simulink model "Senorless"  (R2023a)
settings: Solver=FixedStepDiscrete  StartTime=0.0  StopTime=5  FixedStep=1/FOC_FRQ  RelTol=1e-3
values from neighbouring files (symbols this model uses):
  ADC_REF = 3.6    [Senorless.sldd]
  ADC_SAMPLE_MAX = 32767.0    [Senorless.sldd]
  AMP_GAIN = 16.0    [Senorless.sldd]
  CURR_INPUT = 3276.0    [Senorless.sldd]
  CURR_KI = 380.0    [Senorless.sldd]
  CURR_KP = 0.04    [Senorless.sldd]
  CURR_LIMIT = 0.95    [Senorless.sldd]
  CURR_OVER = 6.0    [Senorless.sldd]
  CURR_POINT_GAIN = 7.0    [Senorless.sldd]
  CURR_STEP = 32760.0    [Senorless.sldd]
  CURR_UNDER = 0.03    [Senorless.sldd]
  CURR_WIDTH = 6552.0    [Senorless.sldd]
  FOC_FRQ = 25000.0    [Senorless.sldd]
  GAMMA = 32767.0    [Senorless.sldd]
  IMAX = 10.0    [Senorless.sldd]
  LPF_FRQ = 2000.0    [Senorless.sldd]
  MOTOR_DAMPER = 2.06E-7    [Senorless.sldd]
  MOTOR_FLUX = 0.00212352    [Senorless.sldd]
  MOTOR_INERTIA = 4.0E-7    [Senorless.sldd]
  MOTOR_LS = 0.000536    [Senorless.sldd]
  MOTOR_PN = 7.0    [Senorless.sldd]
  MOTOR_RS = 4.0    [Senorless.sldd]
  OPEN_IQ = 0.28    [Senorless.sldd]
  OPEN_IQ_MIN = 0.05    [Senorless.sldd]
  OPEN_IQ_SLOW = 0.1    [Senorless.sldd]
  OPEN_SPD = 1000.0    [Senorless.sldd]
  OPEN_SPD_SLOW = 180.0    [Senorless.sldd]
  OPEN_TIME = 0.5    [Senorless.sldd]
  OPEN_TIME_NFO = 0.5    [Senorless.sldd]
  PLL_LIMIT = 0.9    [Senorless.sldd]
  PLL_WIDTH = 800.0    [Senorless.sldd]
  PWM_FRQ = 96000000.0    [Senorless.sldd]
  RS_HUNT = 0.02    [Senorless.sldd]
  SMOK_FRQ = 600.0    [Senorless.sldd]
  SPD_LIMIT = 0.9    [Senorless.sldd]
  SPD_LPF_LEVEL = 0.0    [Senorless.sldd]
  SPD_MAX = 12000.0    [Senorless.sldd]
  SPD_MIN = 4000.0    [Senorless.sldd]
  SPD_REDUCE = 380.0    [Senorless.sldd]
  SPD_STEP = 6.0    [Senorless.sldd]
  SPD_WIDTH = 20.0    [Senorless.sldd]
  THETA_ERR_LIMIT = 8192.0    [Senorless.sldd]
  TS_POINT_GAIN = 10.0    [Senorless.sldd]
  UDC = 48.0    [Senorless.sldd]
  UDC_GAIN = 21.0    [Senorless.sldd]
  UDC_POINT_GAIN = 10.0    [Senorless.sldd]
undefined symbols (not defined in the file or in its folder): curr_q_ki, curr_q_kp, DiscIntNeverNeededParam, magnitude, PLL_LPF_LEVEL, Udc
libraries: simulink x20, slpidlib x5, mcbcontrolslib x2, mcbplantlib x1, autolibpmsmexterior x1, spspowerguiLib x1
(part 4 of 8)

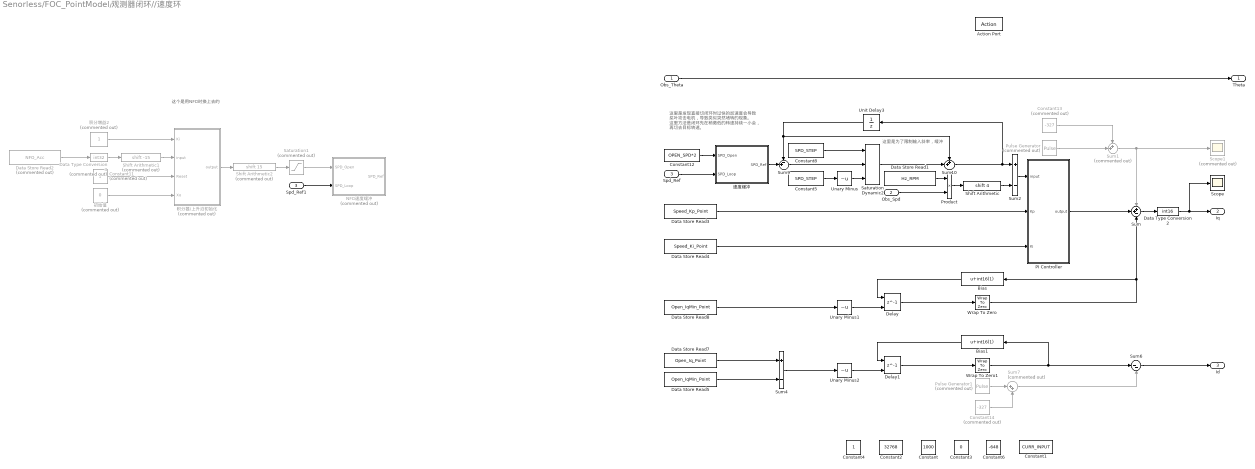
== system Senorless/FOC_PointModel/观测器闭环//速度环 ==
  note: 这个是用NFO时换上去的
  note: 这里是发现直接切闭环时过快的加速度会导致
      | 桨叶攻击电机，导致类似突然堵转的现象。
      | 这里方法是闭环先在稍微低的转速持续一小会，
      | 再切去目标转速。
  note: 这里是为了限制输入斜率，缓冲
  Obs_Theta : Inport
  Obs_Spd : Inport  Port=2
  Spd_Ref : Inport  Port=3
  Action Port : ActionPort  InitializeStates=reset  ActionPortLabel=case [ 4 ]:
  Bias : Bias  Bias=int16(1)  SaturateOnIntegerOverflow=off
  Bias1 : Bias  Bias=int16(1)  SaturateOnIntegerOverflow=off
  Constant : Constant  Value=1000  OutDataTypeStr=int16
  Constant1 : Constant  Value=CURR_INPUT  OutDataTypeStr=int16
  Constant11 : Constant  Commented=on  OutDataTypeStr=uint8
  Constant12 : Constant  Value=OPEN_SPD*2  OutDataTypeStr=int32
  Constant13 : Constant  Commented=on  Value=-327  OutDataTypeStr=int32
  Constant14 : Constant  Commented=on  Value=-327  OutDataTypeStr=int16
  Constant2 : Constant  Value=32768  OutDataTypeStr=int16
  Constant3 : Constant  Value=0  OutDataTypeStr=int16
  Constant4 : Constant  OutDataTypeStr=int16
  Constant5 : Constant  Value=SPD_STEP  OutDataTypeStr=int32
  Constant6 : Constant  Value=-648  OutDataTypeStr=int16
  Constant8 : Constant  Value=SPD_STEP  OutDataTypeStr=int32
  Data Store Read1 : DataStoreRead  DataStoreName=Hz_RPM  IndexOptions=Index vector (dialog)  Indices=1  OutputSizes=1
  Data Store Read2 : DataStoreRead  Commented=on  DataStoreName=NFO_Acc  IndexOptions=Index vector (dialog)  Indices=1  OutputSizes=1
  Data Store Read3 : DataStoreRead  DataStoreName=Speed_Kp_Point  IndexOptions=Index vector (dialog)  Indices=1  OutputSizes=1
  Data Store Read4 : DataStoreRead  DataStoreName=Speed_Ki_Point  IndexOptions=Index vector (dialog)  Indices=1  OutputSizes=1
  Data Store Read5 : DataStoreRead  DataStoreName=Open_IqMin_Point  IndexOptions=Index vector (dialog)  Indices=1  OutputSizes=1
  Data Store Read7 : DataStoreRead  DataStoreName=Open_Iq_Point  IndexOptions=Index vector (dialog)  Indices=1  OutputSizes=1
  Data Store Read8 : DataStoreRead  DataStoreName=Open_IqMin_Point  IndexOptions=Index vector (dialog)  Indices=1  OutputSizes=1
  Data Type Conversion2 : DataTypeConversion  OutDataTypeStr=int16  SaturateOnIntegerOverflow=off
  Data Type Conversion3 : DataTypeConversion  Commented=on  OutDataTypeStr=int32  SaturateOnIntegerOverflow=off
  Delay : Delay  DelayLength=1  InitialConditionSource=Input port
      settings: InputPortMap=u0,p4
  Delay1 : Delay  DelayLength=1  InitialConditionSource=Input port
      settings: InputPortMap=u0,p4
  NFO速度缓冲 : Stateflow chart  Commented=on  TreatAsAtomicUnit=on
  PI Controller : Subsystem
      settings: MinAlgLoopOccurrences=on
  Product : Product  OutDataTypeStr=int32  RndMeth=Zero
  Pulse Generator : DiscretePulseGenerator  Commented=on  Amplitude=int32(654)  Period=1000  PulseWidth=500  SampleTime=-1
  Pulse Generator1 : DiscretePulseGenerator  Commented=on  Amplitude=int16(327*2)  Period=500  PulseWidth=250  SampleTime=-1
  Saturation Dynamic2 : simulink/Discontinuities/Saturation Dynamic  OutMin=[]  OutMax=[]  OutDataTypeStr=Inherit: Same as second input  OutDataType=fixdt(1, 16)  OutScaling=2^-10  RndMeth=Zero  DoSatur=off
  Saturation1 : Saturate  Commented=on  UpperLimit=SPD_MIN  LowerLimit=0
  Scope : Scope
  Scope1 : Scope  Commented=on
  Shift Arithmetic : ArithShift  BitShiftNumber=4
  Shift Arithmetic1 : ArithShift  Commented=on  BitShiftNumber=-15
  Shift Arithmetic2 : ArithShift  Commented=on  BitShiftNumber=15
  Spd_Ref1 : InportShadow  Port=3
  Sum : Sum  Inputs=++-  RndMeth=Zero
  Sum1 : Sum  Commented=on  Inputs=++|  RndMeth=Zero
  Sum10 : Sum  Inputs=++|  OutDataTypeStr=int32  RndMeth=Zero
  Sum2 : Sum  Inputs=+-  AccumDataTypeStr=int32  OutDataTypeStr=int16  RndMeth=Zero  SaturateOnIntegerOverflow=on
  Sum4 : Sum  Inputs=+-
  Sum6 : Sum  Inputs=|--  OutDataTypeStr=int16  RndMeth=Zero
  Sum7 : Sum  Commented=on  Inputs=|++  RndMeth=Zero
  Sum9 : Sum  Inputs=-+|  AccumDataTypeStr=int16  OutDataTypeStr=int32  RndMeth=Zero
  Unary Minus : UnaryMinus
  Unary Minus1 : UnaryMinus
  Unary Minus2 : UnaryMinus
  Unit Delay3 : UnitDelay  InitialCondition=OPEN_SPD  SampleTime=-1  HasFrameUpgradeWarning=on
  Wrap To Zero : simulink/Discontinuities/Wrap To Zero  Threshold=int16(0)
  Wrap To Zero1 : simulink/Discontinuities/Wrap To Zero  Threshold=int16(0)
  初始值 : Constant  Commented=on  Value=0  OutDataTypeStr=int32
  积分器/上升沿初始化 : Subsystem  Commented=on  TreatAsAtomicUnit=on
      settings: MinAlgLoopOccurrences=on
  积分增益2 : Constant  Commented=on  OutDataTypeStr=int16
  速度缓冲 : Stateflow chart  TreatAsAtomicUnit=on
  Theta : Outport
  Iq : Outport  Port=2
  Id : Outport  Port=3
  wires:
  Obs_Theta/1 -> Theta/1
  Data Store Read4/1 -> PI Controller/3(Ki)
  Data Store Read3/1 -> PI Controller/2(Kp)
  Sum10/1 -> Unit Delay3/1, Sum2/1
  Sum2/1 -> PI Controller/1(input)
  Shift Arithmetic/1 -> Sum2/2
  Data Store Read1/1 -> Product/1
  Obs_Spd/1 -> Product/2
  Saturation Dynamic2/1 -> Sum10/2
  Unit Delay3/1 -> Sum10/1, Sum9/1
  Data Store Read7/1 -> Sum4/1
  Spd_Ref/1 -> 速度缓冲/2(SPD_Loop)
  Product/1 -> Shift Arithmetic/1
  PI Controller/1(output) -> Sum/2
  Sum/1 -> Data Type Conversion2/1
  Constant5/1 -> Unary Minus/1
  积分器/上升沿初始化/1(output) -> Shift Arithmetic2/1
  Data Store Read2/1 -> Data Type Conversion3/1
  积分增益2/1 -> 积分器/上升沿初始化/1(Ki)
  Data Type Conversion3/1 -> Shift Arithmetic1/1
  Shift Arithmetic1/1 -> 积分器/上升沿初始化/2(input)
  Constant12/1 -> 速度缓冲/1(SPD_Open)
  Spd_Ref1/1 -> NFO速度缓冲/2(SPD_Loop)
  Shift Arithmetic2/1 -> Saturation1/1
  Constant11/1 -> 积分器/上升沿初始化/3(Reset)
  初始值/1 -> 积分器/上升沿初始化/4(Xo)
  Saturation1/1 -> NFO速度缓冲/1(SPD_Open)
  速度缓冲/1(SPD_Ref) -> Sum9/2
  Data Store Read5/1 -> Sum4/2
  Data Type Conversion2/1 -> Iq/1, Scope/1
  Sum1/1 -> Sum/1, Scope1/1
  Sum6/1 -> Id/1
  Pulse Generator1/1 -> Sum7/1
  Constant14/1 -> Sum7/2
  Sum7/1 -> Sum6/2
  Sum9/1 -> Saturation Dynamic2/2
  Constant8/1 -> Saturation Dynamic2/1
  Unary Minus/1 -> Saturation Dynamic2/3
  Pulse Generator/1 -> Sum1/2
  Constant13/1 -> Sum1/1
  Sum4/1 -> Unary Minus2/1
  Delay/1 -> Wrap To Zero/1
  Data Store Read8/1 -> Unary Minus1/1
  Unary Minus1/1 -> Delay/2
  Wrap To Zero/1 -> Bias/1, Sum/3
  Unary Minus2/1 -> Delay1/2
  Delay1/1 -> Wrap To Zero1/1
  Wrap To Zero1/1 -> Sum6/1, Bias1/1
  Bias1/1 -> Delay1/1
  Bias/1 -> Delay/1

== system Senorless/FOC_PointModel/预定位 ==
  Action Port : ActionPort  InitializeStates=reset  ActionPortLabel=case [ 1 ]:
  Bias : Bias  Bias=int16(5)  SaturateOnIntegerOverflow=off
  Constant1 : Constant  Value=0  OutDataTypeStr=int16
  Constant2 : Constant  OutDataTypeStr=int16
  Constant3 : Constant  Value=0  OutDataTypeStr=uint16
  Data Store Read3 : DataStoreRead  DataStoreName=Open_Iq_Point  IndexOptions=Index vector (dialog)  Indices=1  OutputSizes=1
  Saturation Dynamic2 : simulink/Discontinuities/Saturation Dynamic  OutMin=[]  OutMax=[]  OutDataTypeStr=Inherit: Same as second input  OutDataType=fixdt(1, 16)  OutScaling=2^-10  RndMeth=Zero  DoSatur=off
  Unit Delay4 : UnitDelay  SampleTime=-1  HasFrameUpgradeWarning=on
  Theta : Outport
  Iq : Outport  Port=2
  Id : Outport  Port=3
  wires:
  Constant3/1 -> Theta/1
  Constant1/1 -> Iq/1
  Saturation Dynamic2/1 -> Unit Delay4/1, Id/1
  Constant2/1 -> Saturation Dynamic2/3
  Bias/1 -> Saturation Dynamic2/2
  Data Store Read3/1 -> Saturation Dynamic2/1
  Unit Delay4/1 -> Bias/1

== system Senorless/FOC_PointModel/Err/PLL_LPF1 ==
  note: y(n)=ax(n)+(1−a)y(n−1)
  note: a =(ω c​ T s​ )/(1+ω c​ T s​ )
  input : Inport
  Constant1 : Constant  Value=15  OutDataTypeStr=int16
  Constant5 : Constant  OutDataTypeStr=int16
  Product10 : Product  OutDataTypeStr=int32
  Product11 : Product  OutDataTypeStr=int32  RndMeth=Zero
  Shift Arithmetic1 : ArithShift  BitShiftNumber=-4
  Shift Arithmetic9 : ArithShift  BitShiftNumber=4
  Sum10 : Sum  Inputs=-+
  Sum11 : Sum  OutDataTypeStr=int32  RndMeth=Zero
  Unit Delay9 : UnitDelay  SampleTime=-1  HasFrameUpgradeWarning=on
  output : Outport
  wires:
  input/1 -> Product10/2
  Unit Delay9/1 -> Product11/1
  Product10/1 -> Sum11/2
  Product11/1 -> Sum11/1
  Sum10/1 -> Product10/1
  Shift Arithmetic1/1 -> Sum10/2
  Shift Arithmetic9/1 -> Unit Delay9/1, output/1
  Sum11/1 -> Shift Arithmetic9/1
  Constant5/1 -> Shift Arithmetic1/1
  Constant1/1 -> Product11/2, Sum10/1

== system Senorless/FOC_PointModel/Err/闭环错误判断 ==
  Curr_Err : Inport
  Curr_Max : Inport  Port=2
  Obs_SPD : Inport  Port=3
  Udc_Ref : Inport  Port=4
  Enable : EnablePort  StatesWhenEnabling=reset
  Constant : Constant  Value=16384  OutDataTypeStr=int32
  Data Store Read : DataStoreRead  DataStoreName=FOC_FRQ_Point  IndexOptions=Index vector (dialog)  Indices=1  OutputSizes=1
  Data Store Read4 : DataStoreRead  DataStoreName=Open_Hz  IndexOptions=Index vector (dialog)  Indices=1  OutputSizes=1
  Data Store Read7 : DataStoreRead  DataStoreName=Curr_Under  IndexOptions=Index vector (dialog)  Indices=1  OutputSizes=1
  Data Type Conversion12 : DataTypeConversion  OutDataTypeStr=int32  SaturateOnIntegerOverflow=off
  Data Type Conversion13 : DataTypeConversion  OutDataTypeStr=uint8  SaturateOnIntegerOverflow=off
  If1 : If
  Logical Operator : Logic  Operator=OR  Inputs=3  AllPortsSameDT=off  OutDataTypeStr=boolean
  Merge3 : Merge
  OR1 : Logic  Operator=OR  AllPortsSameDT=off  OutDataTypeStr=boolean
  Relational Operator1 : RelationalOperator  Operator=<  OutDataTypeStr=boolean  RndMeth=Zero  InputSameDT=off
  Relational Operator2 : RelationalOperator  Operator=<  OutDataTypeStr=boolean  RndMeth=Zero  InputSameDT=off
  Relational Operator3 : RelationalOperator  OutDataTypeStr=boolean  RndMeth=Zero  InputSameDT=off
  Relational Operator4 : RelationalOperator  Operator=<  OutDataTypeStr=boolean  RndMeth=Zero  InputSameDT=off
  SUM : Subsystem
  Scope : Scope
  Scope1 : Scope
  Scope2 : Scope
  Shift Arithmetic1 : ArithShift  BitShiftNumber=1
  Shift Arithmetic3 : ArithShift  BitShiftNumber=1
  Unit Delay : UnitDelay  SampleTime=-1  HasFrameUpgradeWarning=on
  ZERO : Subsystem
  Run_Err : Outport
  wires:
  If1/2 -> ZERO/Action
  Data Store Read/1 -> Shift Arithmetic1/1
  Data Store Read7/1 -> Relational Operator1/2
  Data Type Conversion12/1 -> SUM/1(in)
  Data Store Read4/1 -> Shift Arithmetic3/1
  Logical Operator/1 -> Data Type Conversion12/1, Data Type Conversion13/1
  ZERO/1(out) -> Merge3/2
  Relational Operator3/1 -> Scope2/1, OR1/2
  Curr_Max/1 -> Relational Operator1/1
  Curr_Err/1 -> OR1/1
  If1/1 -> SUM/Action
  Shift Arithmetic3/1 -> Relational Operator2/2
  Merge3/1 -> Scope1/1, Relational Operator3/1
  OR1/1 -> Scope/1, Run_Err/1
  Data Type Conversion13/1 -> If1/1
  SUM/1(out) -> Merge3/1
  Shift Arithmetic1/1 -> Relational Operator3/2
  Relational Operator2/1 -> Logical Operator/3
  Relational Operator1/1 -> Logical Operator/2
  Relational Operator4/1 -> Logical Operator/1
  Constant/1 -> Relational Operator4/2
  Udc_Ref/1 -> Relational Operator4/1
  Obs_SPD/1 -> Unit Delay/1
  Unit Delay/1 -> Relational Operator2/1

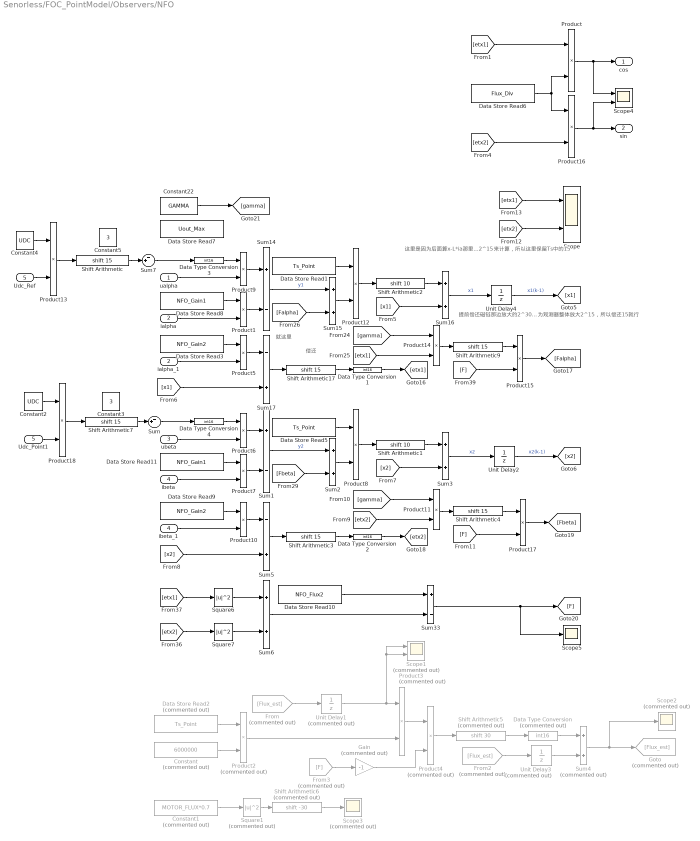
== system Senorless/FOC_PointModel/Observers/NFO ==
  note: 提前偿还磁链那边放大的2^30，因为观测器整体放大2^15，所以偿还15就行
  note: 偿还
  note: 就这里
  note: 这里是因为后面算x-L*ia那里需要再放大2^15来计算，所以这里保留Ts中的15
  ualpha : Inport
  ialpha : Inport  Port=2
  ubeta : Inport  Port=3
  ibeta : Inport  Port=4
  Udc_Ref : Inport  Port=5
  Constant : Constant  Commented=on  Value=6000000  OutDataTypeStr=int32
  Constant1 : Constant  Commented=on  Value=MOTOR_FLUX*0.7  OutDataTypeStr=single
  Constant2 : Constant  Value=UDC  OutDataTypeStr=int16
  Constant22 : Constant  Value=GAMMA  OutDataTypeStr=uint32
  Constant3 : Constant  Value=3  OutDataTypeStr=int16
  Constant4 : Constant  Value=UDC  OutDataTypeStr=int16
  Constant5 : Constant  Value=3  OutDataTypeStr=int16
  Data Store Read1 : DataStoreRead  DataStoreName=Ts_Point  IndexOptions=Index vector (dialog)  Indices=1  OutputSizes=1
  Data Store Read10 : DataStoreRead  DataStoreName=NFO_Flux2  IndexOptions=Index vector (dialog)  Indices=1  OutputSizes=1
  Data Store Read11 : DataStoreRead  DataStoreName=NFO_Gain1  IndexOptions=Index vector (dialog)  Indices=1  OutputSizes=1
  Data Store Read2 : DataStoreRead  Commented=on  DataStoreName=Ts_Point  IndexOptions=Index vector (dialog)  Indices=1  OutputSizes=1
  Data Store Read3 : DataStoreRead  DataStoreName=NFO_Gain2  IndexOptions=Index vector (dialog)  Indices=1  OutputSizes=1
  Data Store Read5 : DataStoreRead  DataStoreName=Ts_Point  IndexOptions=Index vector (dialog)  Indices=1  OutputSizes=1
  Data Store Read6 : DataStoreRead  DataStoreName=Flux_Div  IndexOptions=Index vector (dialog)  Indices=1  OutputSizes=1
  Data Store Read7 : DataStoreRead  DataStoreName=Uout_Max  IndexOptions=Index vector (dialog)  Indices=1  OutputSizes=1
  Data Store Read8 : DataStoreRead  DataStoreName=NFO_Gain1  IndexOptions=Index vector (dialog)  Indices=1  OutputSizes=1
  Data Store Read9 : DataStoreRead  DataStoreName=NFO_Gain2  IndexOptions=Index vector (dialog)  Indices=1  OutputSizes=1
  Data Type Conversion : DataTypeConversion  Commented=on  OutDataTypeStr=int16  SaturateOnIntegerOverflow=off
  Data Type Conversion{1..4} (4 alike) : DataTypeConversion  OutDataTypeStr=int16  SaturateOnIntegerOverflow=off
  From : From  Commented=on  GotoTag=Flux_est
  From2 : From  Commented=on  GotoTag=Flux_est
  From3 : From  Commented=on  GotoTag=F
  Gain : Gain  Commented=on  Gain=-1  OutDataTypeStr=int16  RndMeth=Zero
  Goto : Goto  Commented=on  GotoTag=Flux_est
  Product : Product
  Product{1,5..12,14..15,17} (12 alike) : Product  OutDataTypeStr=int32  RndMeth=Zero
  Product13 : Product  OutDataTypeStr=int32
  Product16 : Product
  Product18 : Product  OutDataTypeStr=int32
  Product2 : Product  Commented=on  OutDataTypeStr=int32  RndMeth=Zero
  Product3 : Product  Commented=on  OutDataTypeStr=int32  RndMeth=Zero
  Product4 : Product  Commented=on  OutDataTypeStr=int32  RndMeth=Zero
  Scope : Scope  NumInputPorts=2
  Scope1 : Scope  Commented=on  NumInputPorts=2
  Scope2 : Scope  Commented=on
  Scope3 : Scope  Commented=on
  Scope4 : Scope  NumInputPorts=2
  Scope5 : Scope
  Shift Arithmetic{,3..4,7,9,17} (6 alike) : ArithShift  BitShiftNumber=15
  Shift Arithmetic1 : ArithShift  BitShiftNumber=10
  Shift Arithmetic2 : ArithShift  BitShiftNumber=10
  Shift Arithmetic5 : ArithShift  Commented=on  BitShiftNumber=30
  Shift Arithmetic6 : ArithShift  Commented=on  BitShiftNumber=-30
  Square1 : Math  Commented=on  Operator=magnitude^2
  Square6 : Math  Operator=magnitude^2
  Square7 : Math  Operator=magnitude^2
  Sum : Sum  Inputs=-+|
  Sum1 : Sum  Inputs=+-  OutDataTypeStr=int32  RndMeth=Zero
  Sum14 : Sum  Inputs=+-  OutDataTypeStr=int32  RndMeth=Zero
  Sum{2..3,6,15..16} (5 alike) : Sum  OutDataTypeStr=int32  RndMeth=Zero
  Sum17 : Sum  Inputs=-+  OutDataTypeStr=int32  RndMeth=Zero
  Sum33 : Sum  Inputs=+-  OutDataTypeStr=int16  RndMeth=Zero
  Sum4 : Sum  Commented=on  OutDataTypeStr=int16  RndMeth=Zero
  Sum5 : Sum  Inputs=-+  OutDataTypeStr=int32  RndMeth=Zero
  Sum7 : Sum  Inputs=-+|
  Udc_Point1 : InportShadow  Port=5
  Unit Delay1 : UnitDelay  Commented=on  SampleTime=-1  HasFrameUpgradeWarning=on
  Unit Delay2 : UnitDelay  SampleTime=-1  HasFrameUpgradeWarning=on
  Unit Delay3 : UnitDelay  Commented=on  InitialCondition=4842  SampleTime=-1  HasFrameUpgradeWarning=on
  Unit Delay4 : UnitDelay  SampleTime=-1  HasFrameUpgradeWarning=on
  ialpha_1 : InportShadow  Port=2
  ibeta_1 : InportShadow  Port=4
  cos : Outport
  sin : Outport  Port=2
  wires:
  Sum3/1 -> Unit Delay2/1  "x2"
  [gamma] -> Product14/1
  Product17/1 -> [Fbeta]
  Unit Delay2/1 -> [x2]  "x2(k-1)"
  Data Store Read1/1 -> Product12/1
  [etx1] -> Scope/1
  [x1] -> Sum16/2
  Data Store Read9/1 -> Product10/1
  ialpha_1/1 -> Product5/2
  Product1/1 -> Sum14/2
  [x2] -> Sum5/2
  Constant22/1 -> [gamma]
  Shift Arithmetic4/1 -> Product17/1
  ubeta/1 -> Product6/2
  Sum6/1 -> Sum33/2
  Sum15/1 -> Product12/2
  Product12/1 -> Shift Arithmetic2/1
  Sum2/1 -> Product8/2
  Product8/1 -> Shift Arithmetic1/1
  [gamma] -> Product11/1
  [x2] -> Sum3/2
  ibeta/1 -> Product7/2
  Square6/1 -> Sum6/1
  Product7/1 -> Sum1/2
  Sum17/1 -> Shift Arithmetic17/1
  Data Store Read5/1 -> Product8/1
  ialpha/1 -> Product1/2
  [etx2] -> Scope/2
  Sum5/1 -> Shift Arithmetic3/1
  ualpha/1 -> Product9/2
  [F] -> Product17/2
  [Falpha] -> Sum15/2
  Product10/1 -> Sum5/1
  Product11/1 -> Shift Arithmetic4/1
  Sum16/1 -> Unit Delay4/1  "x1"
  Product5/1 -> Sum17/1
  Data Store Read8/1 -> Product1/1
  [etx2] -> Square7/1
  [etx2] -> Product11/2
  [Fbeta] -> Sum2/2
  Shift Arithmetic2/1 -> Sum16/1
  Unit Delay4/1 -> [x1]  "x1(k-1)"
  Product15/1 -> [Falpha]
  [etx1] -> Product14/2
  [etx1] -> Square6/1
  Shift Arithmetic3/1 -> Data Type Conversion2/1
  Shift Arithmetic1/1 -> Sum3/1
  [x1] -> Sum17/2
  ibeta_1/1 -> Product10/2
  Data Store Read11/1 -> Product7/1
  Sum14/1 -> Sum15/1  "y1"
  Shift Arithmetic17/1 -> Data Type Conversion1/1
  Sum1/1 -> Sum2/1  "y2"
  Data Store Read3/1 -> Product5/1
  Square7/1 -> Sum6/2
  Constant/1 -> Product2/2
  Data Store Read2/1 -> Product2/1
  Sum33/1 -> Scope5/1, [F]
  From3/1 -> Gain/1
  Product4/1 -> Shift Arithmetic5/1
  Unit Delay1/1 -> Scope1/2, Scope1/1, Product3/1
  From/1 -> Unit Delay1/1
  Product3/1 -> Product4/1
  Shift Arithmetic5/1 -> Data Type Conversion/1
  Gain/1 -> Product4/2
  Data Type Conversion/1 -> Sum4/1
  Unit Delay3/1 -> Sum4/2
  Sum4/1 -> Goto/1, Scope2/1
  From2/1 -> Unit Delay3/1
  Product2/1 -> Product3/2
  Constant1/1 -> Square1/1
  Square1/1 -> Shift Arithmetic6/1
  Shift Arithmetic6/1 -> Scope3/1
  Data Store Read10/1 -> Sum33/1
  Data Store Read6/1 -> Product16/1, Product/2
  Product/1 -> cos/1, Scope4/1
  Product16/1 -> sin/1, Scope4/2
  Product14/1 -> Shift Arithmetic9/1
  Data Type Conversion1/1 -> [etx1]
  Shift Arithmetic9/1 -> Product15/1
  [F] -> Product15/2
  Data Type Conversion2/1 -> [etx2]
  [etx1] -> Product/1
  [etx2] -> Product16/2
  Product13/1 -> Shift Arithmetic/1
  Constant4/1 -> Product13/1
  Udc_Ref/1 -> Product13/2
  Constant2/1 -> Product18/1
  Product18/1 -> Shift Arithmetic7/1
  Udc_Point1/1 -> Product18/2
  Product9/1 -> Sum14/1
  Product6/1 -> Sum1/1
  Data Type Conversion3/1 -> Product9/1
  Shift Arithmetic7/1 -> Sum/2
  Data Type Conversion4/1 -> Product6/1
  Sum/1 -> Data Type Conversion4/1
  Shift Arithmetic/1 -> Sum7/2
  Sum7/1 -> Data Type Conversion3/1

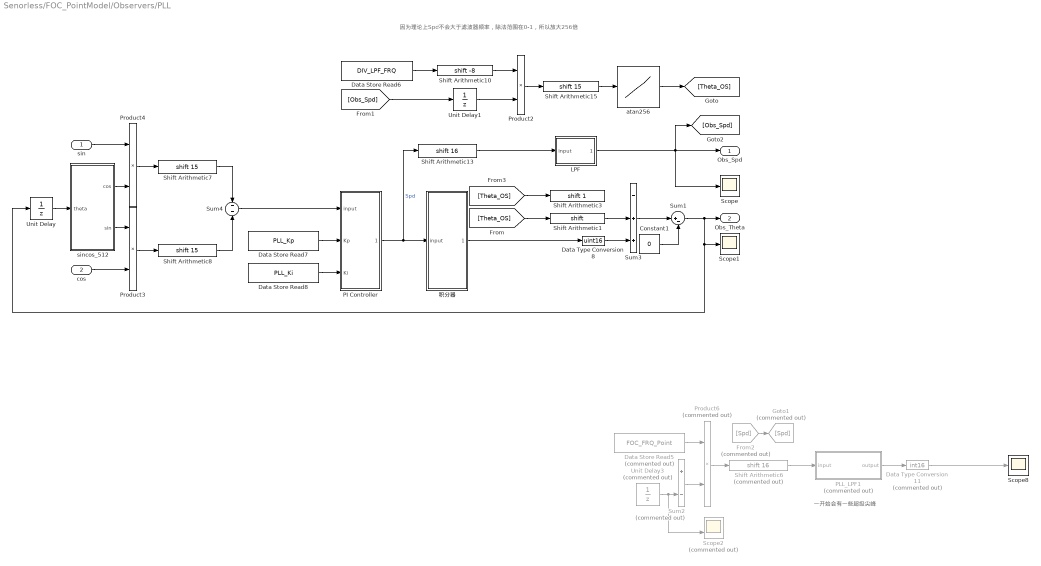
== system Senorless/FOC_PointModel/Observers/PLL ==
  note: 一开始会有一些超级尖峰
  note: 因为理论上Spd不会大于滤波器频率，除法范围在0-1，所以放大256倍
  sin : Inport
  cos : Inport  Port=2
  Constant1 : Constant  Value=0  OutDataTypeStr=uint16
  Data Store Read5 : DataStoreRead  Commented=on  DataStoreName=FOC_FRQ_Point  IndexOptions=Index vector (dialog)  Indices=1  OutputSizes=1
  Data Store Read6 : DataStoreRead  DataStoreName=DIV_LPF_FRQ  IndexOptions=Index vector (dialog)  Indices=1  OutputSizes=1
  Data Store Read7 : DataStoreRead  DataStoreName=PLL_Kp  IndexOptions=Index vector (dialog)  Indices=1  OutputSizes=1
  Data Store Read8 : DataStoreRead  DataStoreName=PLL_Ki  IndexOptions=Index vector (dialog)  Indices=1  OutputSizes=1
  Data Type Conversion11 : DataTypeConversion  Commented=on  OutDataTypeStr=int16  SaturateOnIntegerOverflow=off
  Data Type Conversion8 : DataTypeConversion  OutDataTypeStr=uint16  SaturateOnIntegerOverflow=off
  From2 : From  Commented=on  GotoTag=Spd
  Goto1 : Goto  Commented=on  GotoTag=Spd
  LPF : Subsystem  TreatAsAtomicUnit=on
  PI Controller : Subsystem
      settings: MinAlgLoopOccurrences=on
  PLL_LPF1 : Subsystem  Commented=on  TreatAsAtomicUnit=on
  Product2 : Product  OutDataTypeStr=int32  RndMeth=Zero
  Product3 : Product  OutDataTypeStr=int32  RndMeth=Zero
  Product4 : Product  OutDataTypeStr=int32  RndMeth=Zero
  Product6 : Product  Commented=on  OutDataTypeStr=int32  RndMeth=Zero
  Scope : Scope
  Scope1 : Scope
  Scope2 : Scope  Commented=on  NumInputPorts=2
  Scope8 : Scope
  Shift Arithmetic1 : ArithShift
  Shift Arithmetic10 : ArithShift  BitShiftNumber=-8
  Shift Arithmetic13 : ArithShift  BitShiftNumber=16
  Shift Arithmetic15 : ArithShift  BitShiftNumber=15
  Shift Arithmetic3 : ArithShift  BitShiftNumber=1
  Shift Arithmetic6 : ArithShift  Commented=on  BitShiftNumber=16
  Shift Arithmetic7 : ArithShift  BitShiftNumber=15
  Shift Arithmetic8 : ArithShift  BitShiftNumber=15
  Sum1 : Sum  Inputs=|+-  AccumDataTypeStr=uint16  OutDataTypeStr=uint16  RndMeth=Zero
  Sum2 : Sum  Commented=on  Inputs=+-  OutDataTypeStr=int16  RndMeth=Zero
  Sum3 : Sum  Inputs=-++  AccumDataTypeStr=uint16  OutDataTypeStr=uint16  RndMeth=Zero
  Sum4 : Sum  Inputs=--
  Unit Delay : UnitDelay  SampleTime=-1  HasFrameUpgradeWarning=on
  Unit Delay1 : UnitDelay  SampleTime=-1  HasFrameUpgradeWarning=on
  Unit Delay3 : UnitDelay  Commented=on  SampleTime=-1  HasFrameUpgradeWarning=on
  atan256 : Lookup_n-D  NumberOfTableDimensions=1  BreakpointsSpecification=Even spacing  BreakpointsForDimension1=[-5:5]  UseOneInputPortForAllInputData=on  Table=uint16(16384*atan(linspace(0,1,256)))  TableDataTypeStr=uint16  InterpMethod=Flat  RemoveProtectionInput=on  InternalRulePriority=Speed  OutDataTypeStr=uint16  RndMeth=Zero
  sincos_512 : Subsystem
  积分器 : Subsystem
      settings: MinAlgLoopOccurrences=on
  Obs_Spd : Outport
  Obs_Theta : Outport  Port=2
  wires:
  Data Store Read8/1 -> PI Controller/3(Ki)
  From2/1 -> Goto1/1
  Sum2/1 -> Product6/2
  Unit Delay3/1 -> Scope2/2, Sum2/2
  Product6/1 -> Shift Arithmetic6/1
  Data Store Read5/1 -> Product6/1
  Data Store Read7/1 -> PI Controller/2(Kp)
  积分器/1(output) -> Data Type Conversion8/1
  Shift Arithmetic6/1 -> PLL_LPF1/1(input)
  Sum3/1 -> Sum1/1
  Data Type Conversion8/1 -> Sum3/3
  PI Controller/1(output) -> 积分器/1(input), Shift Arithmetic13/1  "Spd"
  PLL_LPF1/1(output) -> Data Type Conversion11/1
  Data Type Conversion11/1 -> Scope8/1
  [Theta_OS] -> Shift Arithmetic3/1
  [Theta_OS] -> Shift Arithmetic1/1
  Constant1/1 -> Sum1/2
  Shift Arithmetic13/1 -> LPF/1(input)
  LPF/1(output) -> [Obs_Spd], Obs_Spd/1, Scope/1
  Shift Arithmetic1/1 -> Sum3/2
  Shift Arithmetic7/1 -> Sum4/1
  Product4/1 -> Shift Arithmetic7/1
  sin/1 -> Product4/1
  cos/1 -> Product3/2
  sincos_512/1(cos) -> Product4/2
  Shift Arithmetic8/1 -> Sum4/2
  Product3/1 -> Shift Arithmetic8/1
  sincos_512/2(sin) -> Product3/1
  Sum4/1 -> PI Controller/1(input)
  Product2/1 -> Shift Arithmetic15/1
  [Obs_Spd] -> Unit Delay1/1
  Data Store Read6/1 -> Shift Arithmetic10/1
  Unit Delay1/1 -> Product2/2
  atan256/1 -> [Theta_OS]
  Shift Arithmetic15/1 -> atan256/1
  Shift Arithmetic10/1 -> Product2/1
  Sum1/1 -> Obs_Theta/1, Unit Delay/1, Scope1/1
  Unit Delay/1 -> sincos_512/1(theta)

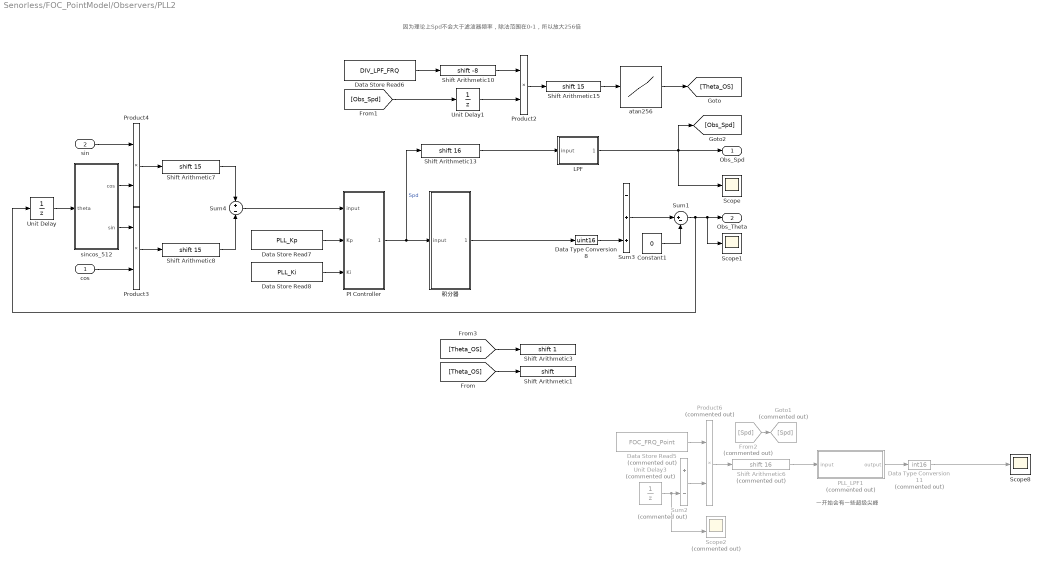
== system Senorless/FOC_PointModel/Observers/PLL2 ==
  note: 因为理论上Spd不会大于滤波器频率，除法范围在0-1，所以放大256倍
  note: 一开始会有一些超级尖峰
  cos : Inport
  sin : Inport  Port=2
  Constant1 : Constant  Value=0  OutDataTypeStr=uint16
  Data Store Read5 : DataStoreRead  Commented=on  DataStoreName=FOC_FRQ_Point  IndexOptions=Index vector (dialog)  Indices=1  OutputSizes=1
  Data Store Read6 : DataStoreRead  DataStoreName=DIV_LPF_FRQ  IndexOptions=Index vector (dialog)  Indices=1  OutputSizes=1
  Data Store Read7 : DataStoreRead  DataStoreName=PLL_Kp  IndexOptions=Index vector (dialog)  Indices=1  OutputSizes=1
  Data Store Read8 : DataStoreRead  DataStoreName=PLL_Ki  IndexOptions=Index vector (dialog)  Indices=1  OutputSizes=1
  Data Type Conversion11 : DataTypeConversion  Commented=on  OutDataTypeStr=int16  SaturateOnIntegerOverflow=off
  Data Type Conversion8 : DataTypeConversion  OutDataTypeStr=uint16  SaturateOnIntegerOverflow=off
  From2 : From  Commented=on  GotoTag=Spd
  Goto1 : Goto  Commented=on  GotoTag=Spd
  LPF : Subsystem  TreatAsAtomicUnit=on
  PI Controller : Subsystem
      settings: MinAlgLoopOccurrences=on
  PLL_LPF1 : Subsystem  Commented=on  TreatAsAtomicUnit=on
  Product2 : Product  OutDataTypeStr=int32  RndMeth=Zero
  Product3 : Product  OutDataTypeStr=int32  RndMeth=Zero
  Product4 : Product  OutDataTypeStr=int32  RndMeth=Zero
  Product6 : Product  Commented=on  OutDataTypeStr=int32  RndMeth=Zero
  Scope : Scope
  Scope1 : Scope
  Scope2 : Scope  Commented=on  NumInputPorts=2
  Scope8 : Scope
  Shift Arithmetic1 : ArithShift
  Shift Arithmetic10 : ArithShift  BitShiftNumber=-8
  Shift Arithmetic13 : ArithShift  BitShiftNumber=16
  Shift Arithmetic15 : ArithShift  BitShiftNumber=15
  Shift Arithmetic3 : ArithShift  BitShiftNumber=1
  Shift Arithmetic6 : ArithShift  Commented=on  BitShiftNumber=16
  Shift Arithmetic7 : ArithShift  BitShiftNumber=15
  Shift Arithmetic8 : ArithShift  BitShiftNumber=15
  Sum1 : Sum  Inputs=|+-  AccumDataTypeStr=uint16  OutDataTypeStr=uint16  RndMeth=Zero
  Sum2 : Sum  Commented=on  Inputs=+-  OutDataTypeStr=int16  RndMeth=Zero
  Sum3 : Sum  Inputs=-++  AccumDataTypeStr=uint16  OutDataTypeStr=uint16  RndMeth=Zero
  Sum4 : Sum  Inputs=+-
  Unit Delay : UnitDelay  SampleTime=-1  HasFrameUpgradeWarning=on
  Unit Delay1 : UnitDelay  SampleTime=-1  HasFrameUpgradeWarning=on
  Unit Delay3 : UnitDelay  Commented=on  SampleTime=-1  HasFrameUpgradeWarning=on
  atan256 : Lookup_n-D  NumberOfTableDimensions=1  BreakpointsSpecification=Even spacing  BreakpointsForDimension1=[-5:5]  UseOneInputPortForAllInputData=on  Table=uint16(16384*atan(linspace(0,1,256)))  TableDataTypeStr=uint16  InterpMethod=Flat  RemoveProtectionInput=on  InternalRulePriority=Speed  OutDataTypeStr=uint16  RndMeth=Zero
  sincos_512 : Subsystem
  积分器 : Subsystem
      settings: MinAlgLoopOccurrences=on
  Obs_Spd : Outport
  Obs_Theta : Outport  Port=2
  wires:
  Sum1/1 -> Unit Delay/1, Scope1/1, Obs_Theta/1
  Shift Arithmetic10/1 -> Product2/1
  Shift Arithmetic15/1 -> atan256/1
  atan256/1 -> [Theta_OS]
  Unit Delay1/1 -> Product2/2
  Data Store Read6/1 -> Shift Arithmetic10/1
  [Obs_Spd] -> Unit Delay1/1
  Product2/1 -> Shift Arithmetic15/1
  Sum4/1 -> PI Controller/1(input)
  sincos_512/2(sin) -> Product3/1
  Product3/1 -> Shift Arithmetic8/1
  Shift Arithmetic8/1 -> Sum4/2
  sincos_512/1(cos) -> Product4/2
  cos/1 -> Product3/2
  sin/1 -> Product4/1
  Product4/1 -> Shift Arithmetic7/1
  Shift Arithmetic7/1 -> Sum4/1
  LPF/1(output) -> Scope/1, Obs_Spd/1, [Obs_Spd]
  Shift Arithmetic13/1 -> LPF/1(input)
  Constant1/1 -> Sum1/2
  [Theta_OS] -> Shift Arithmetic1/1
  [Theta_OS] -> Shift Arithmetic3/1
  Data Type Conversion11/1 -> Scope8/1
  PLL_LPF1/1(output) -> Data Type Conversion11/1
  PI Controller/1(output) -> Shift Arithmetic13/1, 积分器/1(input)  "Spd"
  Data Type Conversion8/1 -> Sum3/3
  Shift Arithmetic6/1 -> PLL_LPF1/1(input)
  积分器/1(output) -> Data Type Conversion8/1
  Data Store Read7/1 -> PI Controller/2(Kp)
  Data Store Read5/1 -> Product6/1
  Product6/1 -> Shift Arithmetic6/1
  Unit Delay3/1 -> Sum2/2, Scope2/2
  Sum2/1 -> Product6/2
  From2/1 -> Goto1/1
  Data Store Read8/1 -> PI Controller/3(Ki)
  Sum3/1 -> Sum1/1
  Unit Delay/1 -> sincos_512/1(theta)

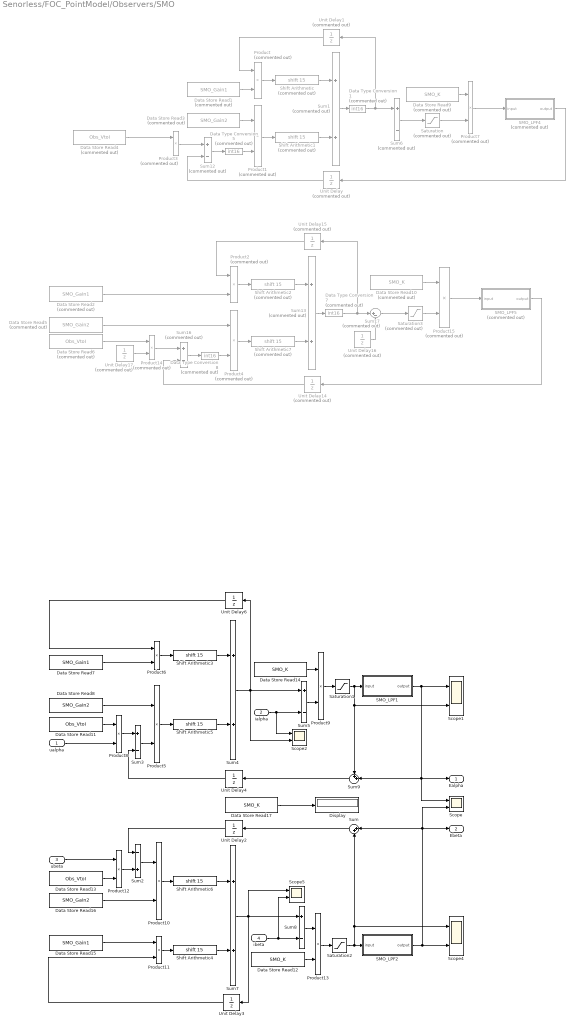
== system Senorless/FOC_PointModel/Observers/SMO ==
  ualpha : Inport
  ialpha : Inport  Port=2
  ubeta : Inport  Port=3
  ibeta : Inport  Port=4
  Data Store Read1 : DataStoreRead  Commented=on  DataStoreName=SMO_Gain1  IndexOptions=Index vector (dialog)  Indices=1  OutputSizes=1
  Data Store Read10 : DataStoreRead  Commented=on  DataStoreName=SMO_K  IndexOptions=Index vector (dialog)  Indices=1  OutputSizes=1
  Data Store Read11 : DataStoreRead  DataStoreName=Obs_VtoI  IndexOptions=Index vector (dialog)  Indices=1  OutputSizes=1
  Data Store Read12 : DataStoreRead  DataStoreName=SMO_K  IndexOptions=Index vector (dialog)  Indices=1  OutputSizes=1
  Data Store Read13 : DataStoreRead  DataStoreName=Obs_VtoI  IndexOptions=Index vector (dialog)  Indices=1  OutputSizes=1
  Data Store Read14 : DataStoreRead  DataStoreName=SMO_K  IndexOptions=Index vector (dialog)  Indices=1  OutputSizes=1
  Data Store Read15 : DataStoreRead  DataStoreName=SMO_Gain1  IndexOptions=Index vector (dialog)  Indices=1  OutputSizes=1
  Data Store Read16 : DataStoreRead  DataStoreName=SMO_Gain2  IndexOptions=Index vector (dialog)  Indices=1  OutputSizes=1
  Data Store Read17 : DataStoreRead  DataStoreName=SMO_K  IndexOptions=Index vector (dialog)  Indices=1  OutputSizes=1
  Data Store Read2 : DataStoreRead  Commented=on  DataStoreName=SMO_Gain1  IndexOptions=Index vector (dialog)  Indices=1  OutputSizes=1
  Data Store Read3 : DataStoreRead  Commented=on  DataStoreName=SMO_Gain2  IndexOptions=Index vector (dialog)  Indices=1  OutputSizes=1
  Data Store Read4 : DataStoreRead  Commented=on  DataStoreName=Obs_VtoI  IndexOptions=Index vector (dialog)  Indices=1  OutputSizes=1
  Data Store Read5 : DataStoreRead  Commented=on  DataStoreName=SMO_Gain2  IndexOptions=Index vector (dialog)  Indices=1  OutputSizes=1
  Data Store Read6 : DataStoreRead  Commented=on  DataStoreName=Obs_VtoI  IndexOptions=Index vector (dialog)  Indices=1  OutputSizes=1
  Data Store Read7 : DataStoreRead  DataStoreName=SMO_Gain1  IndexOptions=Index vector (dialog)  Indices=1  OutputSizes=1
  Data Store Read8 : DataStoreRead  DataStoreName=SMO_Gain2  IndexOptions=Index vector (dialog)  Indices=1  OutputSizes=1
  Data Store Read9 : DataStoreRead  Commented=on  DataStoreName=SMO_K  IndexOptions=Index vector (dialog)  Indices=1  OutputSizes=1
  Data Type Conversion{1,5,7..8} (4 alike) : DataTypeConversion  Commented=on  OutDataTypeStr=int16  SaturateOnIntegerOverflow=off
  Display : Display
  Product{,1..4,7,14..15} (8 alike) : Product  Commented=on  OutDataTypeStr=int32  RndMeth=Zero
  Product{5..6,8..13} (8 alike) : Product  OutDataTypeStr=int32  RndMeth=Zero
  SMO_LPF1 : Subsystem
  SMO_LPF2 : Subsystem
  SMO_LPF4 : Subsystem  Commented=on  TreatAsAtomicUnit=on
  SMO_LPF5 : Subsystem  Commented=on  TreatAsAtomicUnit=on
  Saturation : Saturate  Commented=on  UpperLimit=32768*0.5  LowerLimit=-32768*0.5  OutDataTypeStr=int16  RndMeth=Zero
  Saturation1 : Saturate  UpperLimit=32767  LowerLimit=-32767  OutDataTypeStr=int32  RndMeth=Zero
  Saturation2 : Saturate  UpperLimit=32767  LowerLimit=-32767  OutDataTypeStr=int32  RndMeth=Zero
  Saturation3 : Saturate  Commented=on  UpperLimit=32768*0.5  LowerLimit=-32768*0.5  OutDataTypeStr=int16  RndMeth=Zero
  Scope{,1..2,4..5} (5 alike) : Scope  NumInputPorts=2
  Shift Arithmetic{,1..2,7} (4 alike) : ArithShift  Commented=on  BitShiftNumber=15
  Shift Arithmetic{3..6} (4 alike) : ArithShift  BitShiftNumber=15  DiagnosticForOORShift=Error
  Sum : Sum  Inputs=|++
  Sum1 : Sum  Commented=on
  Sum12 : Sum  Commented=on  Inputs=+-
  Sum13 : Sum  Commented=on
  Sum16 : Sum  Commented=on  Inputs=+-
  Sum17 : Sum  Commented=on  Inputs=|+-  OutDataTypeStr=int16  RndMeth=Zero
  Sum2 : Sum  Inputs=-+
  Sum3 : Sum  Inputs=+-  OutDataTypeStr=int32  RndMeth=Zero
  Sum4 : Sum  OutDataTypeStr=int32  RndMeth=Zero
  Sum5 : Sum  Inputs=+-  OutDataTypeStr=int32  RndMeth=Zero
  Sum6 : Sum  Commented=on  Inputs=+-  OutDataTypeStr=int16  RndMeth=Zero
  Sum7 : Sum  OutDataTypeStr=int32
  Sum8 : Sum  Inputs=+-  OutDataTypeStr=int32  RndMeth=Zero
  Sum9 : Sum  Inputs=++|
  Unit Delay{,1,14..17} (6 alike) : UnitDelay  Commented=on  SampleTime=-1  HasFrameUpgradeWarning=on
  Unit Delay{2..4,6} (4 alike) : UnitDelay  SampleTime=-1  HasFrameUpgradeWarning=on
  Ealpha : Outport
  Ebeta : Outport  Port=2
  wires:
  Shift Arithmetic1/1 -> Sum1/2
  Shift Arithmetic2/1 -> Sum13/1
  Data Store Read1/1 -> Product/2
  Data Store Read4/1 -> Product3/1
  Product1/1 -> Shift Arithmetic1/1
  Product3/1 -> Sum12/1
  Unit Delay/1 -> Sum12/2
  Data Type Conversion1/1 -> Sum6/1, Unit Delay1/1
  Sum1/1 -> Data Type Conversion1/1
  Unit Delay1/1 -> Product/1
  Product/1 -> Shift Arithmetic/1
  Saturation3/1 -> Product15/2
  Data Type Conversion7/1 -> Unit Delay15/1, Sum17/1
  Data Store Read5/1 -> Product4/1
  Saturation/1 -> Product7/2
  Product2/1 -> Shift Arithmetic2/1
  Sum12/1 -> Data Type Conversion5/1
  Sum17/1 -> Saturation3/1
  Data Type Conversion5/1 -> Product1/2
  Unit Delay15/1 -> Product2/1
  Shift Arithmetic/1 -> Sum1/1
  Unit Delay14/1 -> Sum16/2
  Sum13/1 -> Data Type Conversion7/1
  Data Type Conversion8/1 -> Product4/2
  Data Store Read2/1 -> Product2/2
  Shift Arithmetic7/1 -> Sum13/2
  Product4/1 -> Shift Arithmetic7/1
  Unit Delay17/1 -> Product14/2
  Product14/1 -> Sum16/1
  Sum16/1 -> Data Type Conversion8/1
  Data Store Read6/1 -> Product14/1
  Unit Delay16/1 -> Sum17/2
  Data Store Read3/1 -> Product1/1
  Data Store Read9/1 -> Product7/1
  Data Store Read10/1 -> Product15/1
  Product15/1 -> SMO_LPF5/1(input)
  Product7/1 -> SMO_LPF4/1(input)
  SMO_LPF4/1(output) -> Unit Delay/1
  SMO_LPF5/1(output) -> Unit Delay14/1
  Data Store Read7/1 -> Product6/2
  Data Store Read8/1 -> Product5/1
  Product6/1 -> Shift Arithmetic3/1
  Product5/1 -> Shift Arithmetic5/1
  Sum6/1 -> Saturation/1
  Product10/1 -> Shift Arithmetic6/1
  Product11/1 -> Shift Arithmetic4/1
  SMO_LPF1/1(output) -> Ealpha/1, Sum9/2, Scope/1, Scope1/1
  Shift Arithmetic3/1 -> Sum4/1
  Shift Arithmetic5/1 -> Sum4/2
  Sum5/1 -> Product9/2
  Data Store Read17/1 -> Display/1
  Data Store Read14/1 -> Product9/1
  SMO_LPF2/1(output) -> Scope4/2, Scope/2, Ebeta/1, Sum/1
  Sum7/1 -> Scope5/1, Unit Delay3/1, Sum8/1
  Sum4/1 -> Sum5/1, Scope2/2, Unit Delay6/1
  Product9/1 -> Saturation1/1
  Product13/1 -> Saturation2/1
  Sum/1 -> Unit Delay2/1
  Sum9/1 -> Unit Delay4/1
  ialpha/1 -> Scope2/1, Sum5/2
  ibeta/1 -> Scope5/2, Sum8/2
  Unit Delay6/1 -> Product6/1
  Data Store Read11/1 -> Product8/1
  Unit Delay4/1 -> Sum3/2
  Saturation1/1 -> Sum9/1, Scope1/2, SMO_LPF1/1(input)
  Saturation2/1 -> SMO_LPF2/1(input), Scope4/1, Sum/2
  Sum3/1 -> Product5/2
  Product8/1 -> Sum3/1
  ualpha/1 -> Product8/2
  Shift Arithmetic6/1 -> Sum7/1
  Sum2/1 -> Product10/1
  Data Store Read16/1 -> Product10/2
  Product12/1 -> Sum2/2
  Unit Delay2/1 -> Sum2/1
  Shift Arithmetic4/1 -> Sum7/2
  Data Store Read15/1 -> Product11/1
  Unit Delay3/1 -> Product11/2
  Sum8/1 -> Product13/1
  Data Store Read12/1 -> Product13/2
  ubeta/1 -> Product12/1
  Data Store Read13/1 -> Product12/2
